simulink model "Demo_veDYNA_cs"  (Simulink 7.6)
settings: Solver=ode1  StartTime=0  StopTime=15  FixedStep=1/500  RelTol=1e-3
PreLoadFcn:
  | PreScanveDYNAPreLoadFcn(bdroot);
  | check_NUTS_defined;
  | 
  | assignin('base',['model_closed_' bdroot],false);
PostLoadFcn:
  | PreScanveDYNAPostLoadFcn(bdroot);
  | 
InitFcn:
  | vdy_SetExternalInputSource('ManLongCtrl',1,'Brake','other');
  | vdy_SetExternalInputSource('ManLongCtrl',1,'EngineTorque','other');
  | vdy_SetExternalInputSource('ManLatCtrl',1,'Steering','other');
  | 
  | PreScanveDYNAInitFcn(bdroot);
  | PreScanExperimentInitFcn(bdroot)
StopFcn:
  | PreScanExperimentStopFcn(bdroot)
undefined symbols (not defined in the file): at_period, CPT, vm_at_pulsewidth, vm_driver_dflt_gain, x_ini_VRML, y_ini_VRML, z_ini_VRML
libraries: dyna_cpt_lib x93, simulink x16, simulink_extras x14, PreScanSimulinkLibrary x6, anilib x3, dyna_lib x3, dyna_manctrl_lib x2, dyna_road_lib x2, PreScanUsefulBlocks x1, dyna_io_lib x1, dyna_demo_lib x1, dyna_usr_maneuver_states_lib x1
(part 7 of 8)

== system Demo_veDYNA_cs/Vedyna_Vehicle/CPT_MDL/MDL_PAR/Driver/System Instance 1/front_stiff [N/rad] ==
  Table : Lookup  InputValues=CPT.MDL_PAR.Driver{1}.front_stiff.Table.x  Table=CPT.MDL_PAR.Driver{1}.front_stiff.Table.v  SaturateOnIntegerOverflow=on
  Terminator : Terminator
  Terminator1 : Terminator
  Value : Constant  Value=CPT.MDL_PAR.Driver{1}.front_stiff.Value.v
  tag scope: Driver_1_front_stiff_TBL=global, Driver_1_front_stiff_VAL=global
  wires:
  [vdy_Simctrl_tsim] -> Table/1
  Value/1 -> [Driver_1_front_stiff_VAL]
  [Driver_1_front_stiff_VAL] -> Terminator/1
  [Driver_1_front_stiff_TBL] -> Terminator1/1
  Table/1 -> [Driver_1_front_stiff_TBL]

== system Demo_veDYNA_cs/Vedyna_Vehicle/CPT_MDL/MDL_PAR/Driver/System Instance 1/front_stiff_sw [-] ==
  Table : Lookup  InputValues=CPT.MDL_PAR.Driver{1}.front_stiff_sw.Table.x  Table=CPT.MDL_PAR.Driver{1}.front_stiff_sw.Table.v  SaturateOnIntegerOverflow=on
  Terminator : Terminator
  Terminator1 : Terminator
  Value : Constant  Value=CPT.MDL_PAR.Driver{1}.front_stiff_sw.Value.v
  tag scope: Driver_1_front_stiff_sw_TBL=global, Driver_1_front_stiff_sw_VAL=global
  wires:
  [vdy_Simctrl_tsim] -> Table/1
  Value/1 -> [Driver_1_front_stiff_sw_VAL]
  [Driver_1_front_stiff_sw_VAL] -> Terminator/1
  [Driver_1_front_stiff_sw_TBL] -> Terminator1/1
  Table/1 -> [Driver_1_front_stiff_sw_TBL]

== system Demo_veDYNA_cs/Vedyna_Vehicle/CPT_MDL/MDL_PAR/Driver/System Instance 1/gain_lat [-] ==
  Table : Lookup  InputValues=CPT.MDL_PAR.Driver{1}.gain_lat.Table.x  Table=CPT.MDL_PAR.Driver{1}.gain_lat.Table.v  SaturateOnIntegerOverflow=on
  Terminator : Terminator
  Terminator1 : Terminator
  Value : Constant  Value=CPT.MDL_PAR.Driver{1}.gain_lat.Value.v
  tag scope: Driver_1_gain_lat_TBL=global, Driver_1_gain_lat_VAL=global
  wires:
  [vdy_Simctrl_tsim] -> Table/1
  Value/1 -> [Driver_1_gain_lat_VAL]
  [Driver_1_gain_lat_VAL] -> Terminator/1
  [Driver_1_gain_lat_TBL] -> Terminator1/1
  Table/1 -> [Driver_1_gain_lat_TBL]

== system Demo_veDYNA_cs/Vedyna_Vehicle/CPT_MDL/MDL_PAR/Driver/System Instance 1/gain_long [-] ==
  Table : Lookup  InputValues=CPT.MDL_PAR.Driver{1}.gain_long.Table.x  Table=CPT.MDL_PAR.Driver{1}.gain_long.Table.v  SaturateOnIntegerOverflow=on
  Terminator : Terminator
  Terminator1 : Terminator
  Value : Constant  Value=CPT.MDL_PAR.Driver{1}.gain_long.Value.v
  tag scope: Driver_1_gain_long_TBL=global, Driver_1_gain_long_VAL=global
  wires:
  [vdy_Simctrl_tsim] -> Table/1
  Value/1 -> [Driver_1_gain_long_VAL]
  [Driver_1_gain_long_VAL] -> Terminator/1
  [Driver_1_gain_long_TBL] -> Terminator1/1
  Table/1 -> [Driver_1_gain_long_TBL]

== system Demo_veDYNA_cs/Vedyna_Vehicle/CPT_MDL/MDL_PAR/Driver/System Instance 1/lat_for_r_scale [-] ==
  Table : Lookup  InputValues=CPT.MDL_PAR.Driver{1}.lat_for_r_scale.Table.x  Table=CPT.MDL_PAR.Driver{1}.lat_for_r_scale.Table.v  SaturateOnIntegerOverflow=on
  Terminator : Terminator
  Terminator1 : Terminator
  Value : Constant  Value=CPT.MDL_PAR.Driver{1}.lat_for_r_scale.Value.v
  tag scope: Driver_1_lat_for_r_scale_TBL=global, Driver_1_lat_for_r_scale_VAL=global
  wires:
  [vdy_Simctrl_tsim] -> Table/1
  Value/1 -> [Driver_1_lat_for_r_scale_VAL]
  [Driver_1_lat_for_r_scale_VAL] -> Terminator/1
  [Driver_1_lat_for_r_scale_TBL] -> Terminator1/1
  Table/1 -> [Driver_1_lat_for_r_scale_TBL]

== system Demo_veDYNA_cs/Vedyna_Vehicle/CPT_MDL/MDL_PAR/Driver/System Instance 1/lat_for_r_smooth_t [s] ==
  Table : Lookup  InputValues=CPT.MDL_PAR.Driver{1}.lat_for_r_smooth_t.Table.x  Table=CPT.MDL_PAR.Driver{1}.lat_for_r_smooth_t.Table.v  SaturateOnIntegerOverflow=on
  Terminator : Terminator
  Terminator1 : Terminator
  Value : Constant  Value=CPT.MDL_PAR.Driver{1}.lat_for_r_smooth_t.Value.v
  tag scope: Driver_1_lat_for_r_smooth_t_TBL=global, Driver_1_lat_for_r_smooth_t_VAL=global
  wires:
  [vdy_Simctrl_tsim] -> Table/1
  Value/1 -> [Driver_1_lat_for_r_smooth_t_VAL]
  [Driver_1_lat_for_r_smooth_t_VAL] -> Terminator/1
  [Driver_1_lat_for_r_smooth_t_TBL] -> Terminator1/1
  Table/1 -> [Driver_1_lat_for_r_smooth_t_TBL]

== system Demo_veDYNA_cs/Vedyna_Vehicle/CPT_MDL/MDL_PAR/Driver/System Instance 1/lat_for_r_sw [-] ==
  Table : Lookup  InputValues=CPT.MDL_PAR.Driver{1}.lat_for_r_sw.Table.x  Table=CPT.MDL_PAR.Driver{1}.lat_for_r_sw.Table.v  SaturateOnIntegerOverflow=on
  Terminator : Terminator
  Terminator1 : Terminator
  Value : Constant  Value=CPT.MDL_PAR.Driver{1}.lat_for_r_sw.Value.v
  tag scope: Driver_1_lat_for_r_sw_TBL=global, Driver_1_lat_for_r_sw_VAL=global
  wires:
  [vdy_Simctrl_tsim] -> Table/1
  Value/1 -> [Driver_1_lat_for_r_sw_VAL]
  [Driver_1_lat_for_r_sw_VAL] -> Terminator/1
  [Driver_1_lat_for_r_sw_TBL] -> Terminator1/1
  Table/1 -> [Driver_1_lat_for_r_sw_TBL]

== system Demo_veDYNA_cs/Vedyna_Vehicle/CPT_MDL/MDL_PAR/Driver/System Instance 1/path_v_scale [-] ==
  Table : Lookup  InputValues=CPT.MDL_PAR.Driver{1}.path_v_scale.Table.x  Table=CPT.MDL_PAR.Driver{1}.path_v_scale.Table.v  SaturateOnIntegerOverflow=on
  Terminator : Terminator
  Terminator1 : Terminator
  Value : Constant  Value=CPT.MDL_PAR.Driver{1}.path_v_scale.Value.v
  tag scope: Driver_1_path_v_scale_TBL=global, Driver_1_path_v_scale_VAL=global
  wires:
  [vdy_Simctrl_tsim] -> Table/1
  Value/1 -> [Driver_1_path_v_scale_VAL]
  [Driver_1_path_v_scale_VAL] -> Terminator/1
  [Driver_1_path_v_scale_TBL] -> Terminator1/1
  Table/1 -> [Driver_1_path_v_scale_TBL]

== system Demo_veDYNA_cs/Vedyna_Vehicle/CPT_MDL/MDL_PAR/Driver/System Instance 1/path_x_offset [m] ==
  Table : Lookup  InputValues=CPT.MDL_PAR.Driver{1}.path_x_offset.Table.x  Table=CPT.MDL_PAR.Driver{1}.path_x_offset.Table.v  SaturateOnIntegerOverflow=on
  Terminator : Terminator
  Terminator1 : Terminator
  Value : Constant  Value=CPT.MDL_PAR.Driver{1}.path_x_offset.Value.v
  tag scope: Driver_1_path_x_offset_TBL=global, Driver_1_path_x_offset_VAL=global
  wires:
  [vdy_Simctrl_tsim] -> Table/1
  Value/1 -> [Driver_1_path_x_offset_VAL]
  [Driver_1_path_x_offset_VAL] -> Terminator/1
  [Driver_1_path_x_offset_TBL] -> Terminator1/1
  Table/1 -> [Driver_1_path_x_offset_TBL]

== system Demo_veDYNA_cs/Vedyna_Vehicle/CPT_MDL/MDL_PAR/Driver/System Instance 1/psi_path [rad] ==
  Table : Lookup  InputValues=CPT.MDL_PAR.Driver{1}.psi_path.Table.x  Table=CPT.MDL_PAR.Driver{1}.psi_path.Table.v  SaturateOnIntegerOverflow=on
  Terminator : Terminator
  Terminator1 : Terminator
  Value : Constant  Value=CPT.MDL_PAR.Driver{1}.psi_path.Value.v
  tag scope: Driver_1_psi_path_TBL=global, Driver_1_psi_path_VAL=global
  wires:
  [vdy_Driver_s] -> Table/1
  Value/1 -> [Driver_1_psi_path_VAL]
  [Driver_1_psi_path_VAL] -> Terminator/1
  [Driver_1_psi_path_TBL] -> Terminator1/1
  Table/1 -> [Driver_1_psi_path_TBL]

== system Demo_veDYNA_cs/Vedyna_Vehicle/CPT_MDL/MDL_PAR/Driver/System Instance 1/q_path [m] ==
  Table : Lookup  InputValues=CPT.MDL_PAR.Driver{1}.q_path.Table.x  Table=CPT.MDL_PAR.Driver{1}.q_path.Table.v  SaturateOnIntegerOverflow=on
  Terminator : Terminator
  Terminator1 : Terminator
  Value : Constant  Value=CPT.MDL_PAR.Driver{1}.q_path.Value.v
  tag scope: Driver_1_q_path_TBL=global, Driver_1_q_path_VAL=global
  wires:
  [vdy_Driver_s] -> Table/1
  Value/1 -> [Driver_1_q_path_VAL]
  [Driver_1_q_path_VAL] -> Terminator/1
  [Driver_1_q_path_TBL] -> Terminator1/1
  Table/1 -> [Driver_1_q_path_TBL]

== system Demo_veDYNA_cs/Vedyna_Vehicle/CPT_MDL/MDL_PAR/Driver/System Instance 1/rear_stiff [N/rad] ==
  Table : Lookup  InputValues=CPT.MDL_PAR.Driver{1}.rear_stiff.Table.x  Table=CPT.MDL_PAR.Driver{1}.rear_stiff.Table.v  SaturateOnIntegerOverflow=on
  Terminator : Terminator
  Terminator1 : Terminator
  Value : Constant  Value=CPT.MDL_PAR.Driver{1}.rear_stiff.Value.v
  tag scope: Driver_1_rear_stiff_TBL=global, Driver_1_rear_stiff_VAL=global
  wires:
  [vdy_Simctrl_tsim] -> Table/1
  Value/1 -> [Driver_1_rear_stiff_VAL]
  [Driver_1_rear_stiff_VAL] -> Terminator/1
  [Driver_1_rear_stiff_TBL] -> Terminator1/1
  Table/1 -> [Driver_1_rear_stiff_TBL]

== system Demo_veDYNA_cs/Vedyna_Vehicle/CPT_MDL/MDL_PAR/Driver/System Instance 1/rear_stiff_sw [-] ==
  Table : Lookup  InputValues=CPT.MDL_PAR.Driver{1}.rear_stiff_sw.Table.x  Table=CPT.MDL_PAR.Driver{1}.rear_stiff_sw.Table.v  SaturateOnIntegerOverflow=on
  Terminator : Terminator
  Terminator1 : Terminator
  Value : Constant  Value=CPT.MDL_PAR.Driver{1}.rear_stiff_sw.Value.v
  tag scope: Driver_1_rear_stiff_sw_TBL=global, Driver_1_rear_stiff_sw_VAL=global
  wires:
  [vdy_Simctrl_tsim] -> Table/1
  Value/1 -> [Driver_1_rear_stiff_sw_VAL]
  [Driver_1_rear_stiff_sw_VAL] -> Terminator/1
  [Driver_1_rear_stiff_sw_TBL] -> Terminator1/1
  Table/1 -> [Driver_1_rear_stiff_sw_TBL]

== system Demo_veDYNA_cs/Vedyna_Vehicle/CPT_MDL/MDL_PAR/Driver/System Instance 1/steer_max [deg] ==
  Table : Lookup  InputValues=CPT.MDL_PAR.Driver{1}.steer_max.Table.x  Table=CPT.MDL_PAR.Driver{1}.steer_max.Table.v  SaturateOnIntegerOverflow=on
  Terminator : Terminator
  Terminator1 : Terminator
  Value : Constant  Value=CPT.MDL_PAR.Driver{1}.steer_max.Value.v
  tag scope: Driver_1_steer_max_TBL=global, Driver_1_steer_max_VAL=global
  wires:
  [vdy_Simctrl_tsim] -> Table/1
  Value/1 -> [Driver_1_steer_max_VAL]
  [Driver_1_steer_max_VAL] -> Terminator/1
  [Driver_1_steer_max_TBL] -> Terminator1/1
  Table/1 -> [Driver_1_steer_max_TBL]

== system Demo_veDYNA_cs/Vedyna_Vehicle/CPT_MDL/MDL_PAR/Driver/System Instance 1/steer_min [deg] ==
  Table : Lookup  InputValues=CPT.MDL_PAR.Driver{1}.steer_min.Table.x  Table=CPT.MDL_PAR.Driver{1}.steer_min.Table.v  SaturateOnIntegerOverflow=on
  Terminator : Terminator
  Terminator1 : Terminator
  Value : Constant  Value=CPT.MDL_PAR.Driver{1}.steer_min.Value.v
  tag scope: Driver_1_steer_min_TBL=global, Driver_1_steer_min_VAL=global
  wires:
  [vdy_Simctrl_tsim] -> Table/1
  Value/1 -> [Driver_1_steer_min_VAL]
  [Driver_1_steer_min_VAL] -> Terminator/1
  [Driver_1_steer_min_TBL] -> Terminator1/1
  Table/1 -> [Driver_1_steer_min_TBL]

== system Demo_veDYNA_cs/Vedyna_Vehicle/CPT_MDL/MDL_PAR/Driver/System Instance 1/steer_rate_max [deg/s] ==
  Table : Lookup  InputValues=CPT.MDL_PAR.Driver{1}.steer_rate_max.Table.x  Table=CPT.MDL_PAR.Driver{1}.steer_rate_max.Table.v  SaturateOnIntegerOverflow=on
  Terminator : Terminator
  Terminator1 : Terminator
  Value : Constant  Value=CPT.MDL_PAR.Driver{1}.steer_rate_max.Value.v
  tag scope: Driver_1_steer_rate_max_TBL=global, Driver_1_steer_rate_max_VAL=global
  wires:
  [vdy_Simctrl_tsim] -> Table/1
  Value/1 -> [Driver_1_steer_rate_max_VAL]
  [Driver_1_steer_rate_max_VAL] -> Terminator/1
  [Driver_1_steer_rate_max_TBL] -> Terminator1/1
  Table/1 -> [Driver_1_steer_rate_max_TBL]

== system Demo_veDYNA_cs/Vedyna_Vehicle/CPT_MDL/MDL_PAR/Driver/System Instance 1/steer_rate_min [deg/s] ==
  Table : Lookup  InputValues=CPT.MDL_PAR.Driver{1}.steer_rate_min.Table.x  Table=CPT.MDL_PAR.Driver{1}.steer_rate_min.Table.v  SaturateOnIntegerOverflow=on
  Terminator : Terminator
  Terminator1 : Terminator
  Value : Constant  Value=CPT.MDL_PAR.Driver{1}.steer_rate_min.Value.v
  tag scope: Driver_1_steer_rate_min_TBL=global, Driver_1_steer_rate_min_VAL=global
  wires:
  [vdy_Simctrl_tsim] -> Table/1
  Value/1 -> [Driver_1_steer_rate_min_VAL]
  [Driver_1_steer_rate_min_VAL] -> Terminator/1
  [Driver_1_steer_rate_min_TBL] -> Terminator1/1
  Table/1 -> [Driver_1_steer_rate_min_TBL]

== system Demo_veDYNA_cs/Vedyna_Vehicle/CPT_MDL/MDL_PAR/Driver/System Instance 1/steer_smooth_t [s] ==
  Table : Lookup  InputValues=CPT.MDL_PAR.Driver{1}.steer_smooth_t.Table.x  Table=CPT.MDL_PAR.Driver{1}.steer_smooth_t.Table.v  SaturateOnIntegerOverflow=on
  Terminator : Terminator
  Terminator1 : Terminator
  Value : Constant  Value=CPT.MDL_PAR.Driver{1}.steer_smooth_t.Value.v
  tag scope: Driver_1_steer_smooth_t_TBL=global, Driver_1_steer_smooth_t_VAL=global
  wires:
  [vdy_Simctrl_tsim] -> Table/1
  Value/1 -> [Driver_1_steer_smooth_t_VAL]
  [Driver_1_steer_smooth_t_VAL] -> Terminator/1
  [Driver_1_steer_smooth_t_TBL] -> Terminator1/1
  Table/1 -> [Driver_1_steer_smooth_t_TBL]

== system Demo_veDYNA_cs/Vedyna_Vehicle/CPT_MDL/MDL_PAR/Driver/System Instance 1/target_aim_x [m] ==
  Table : Lookup  InputValues=CPT.MDL_PAR.Driver{1}.target_aim_x.Table.x  Table=CPT.MDL_PAR.Driver{1}.target_aim_x.Table.v  SaturateOnIntegerOverflow=on
  Terminator : Terminator
  Terminator1 : Terminator
  Value : Constant  Value=CPT.MDL_PAR.Driver{1}.target_aim_x.Value.v
  tag scope: Driver_1_target_aim_x_TBL=global, Driver_1_target_aim_x_VAL=global
  wires:
  [vdy_Simctrl_tsim] -> Table/1
  Value/1 -> [Driver_1_target_aim_x_VAL]
  [Driver_1_target_aim_x_VAL] -> Terminator/1
  [Driver_1_target_aim_x_TBL] -> Terminator1/1
  Table/1 -> [Driver_1_target_aim_x_TBL]

== system Demo_veDYNA_cs/Vedyna_Vehicle/CPT_MDL/MDL_PAR/Driver/System Instance 1/tgt_a_max [m/s^2] ==
  Table : Lookup  InputValues=CPT.MDL_PAR.Driver{1}.tgt_a_max.Table.x  Table=CPT.MDL_PAR.Driver{1}.tgt_a_max.Table.v  SaturateOnIntegerOverflow=on
  Terminator : Terminator
  Terminator1 : Terminator
  Value : Constant  Value=CPT.MDL_PAR.Driver{1}.tgt_a_max.Value.v
  tag scope: Driver_1_tgt_a_max_TBL=global, Driver_1_tgt_a_max_VAL=global
  wires:
  [vdy_Simctrl_tsim] -> Table/1
  Value/1 -> [Driver_1_tgt_a_max_VAL]
  [Driver_1_tgt_a_max_VAL] -> Terminator/1
  [Driver_1_tgt_a_max_TBL] -> Terminator1/1
  Table/1 -> [Driver_1_tgt_a_max_TBL]

== system Demo_veDYNA_cs/Vedyna_Vehicle/CPT_MDL/MDL_PAR/Driver/System Instance 1/tgt_acc_smooth_t [s] ==
  Table : Lookup  InputValues=CPT.MDL_PAR.Driver{1}.tgt_acc_smooth_t.Table.x  Table=CPT.MDL_PAR.Driver{1}.tgt_acc_smooth_t.Table.v  SaturateOnIntegerOverflow=on
  Terminator : Terminator
  Terminator1 : Terminator
  Value : Constant  Value=CPT.MDL_PAR.Driver{1}.tgt_acc_smooth_t.Value.v
  tag scope: Driver_1_tgt_acc_smooth_t_TBL=global, Driver_1_tgt_acc_smooth_t_VAL=global
  wires:
  [vdy_Simctrl_tsim] -> Table/1
  Value/1 -> [Driver_1_tgt_acc_smooth_t_VAL]
  [Driver_1_tgt_acc_smooth_t_VAL] -> Terminator/1
  [Driver_1_tgt_acc_smooth_t_TBL] -> Terminator1/1
  Table/1 -> [Driver_1_tgt_acc_smooth_t_TBL]

== system Demo_veDYNA_cs/Vedyna_Vehicle/CPT_MDL/MDL_PAR/Driver/System Instance 1/tgt_ax_max [m/s^2] ==
  Table : Lookup  InputValues=CPT.MDL_PAR.Driver{1}.tgt_ax_max.Table.x  Table=CPT.MDL_PAR.Driver{1}.tgt_ax_max.Table.v  SaturateOnIntegerOverflow=on
  Terminator : Terminator
  Terminator1 : Terminator
  Value : Constant  Value=CPT.MDL_PAR.Driver{1}.tgt_ax_max.Value.v
  tag scope: Driver_1_tgt_ax_max_TBL=global, Driver_1_tgt_ax_max_VAL=global
  wires:
  [vdy_Simctrl_tsim] -> Table/1
  Value/1 -> [Driver_1_tgt_ax_max_VAL]
  [Driver_1_tgt_ax_max_VAL] -> Terminator/1
  [Driver_1_tgt_ax_max_TBL] -> Terminator1/1
  Table/1 -> [Driver_1_tgt_ax_max_TBL]

== system Demo_veDYNA_cs/Vedyna_Vehicle/CPT_MDL/MDL_PAR/Driver/System Instance 1/tgt_ax_min [m/s^2] ==
  Table : Lookup  InputValues=CPT.MDL_PAR.Driver{1}.tgt_ax_min.Table.x  Table=CPT.MDL_PAR.Driver{1}.tgt_ax_min.Table.v  SaturateOnIntegerOverflow=on
  Terminator : Terminator
  Terminator1 : Terminator
  Value : Constant  Value=CPT.MDL_PAR.Driver{1}.tgt_ax_min.Value.v
  tag scope: Driver_1_tgt_ax_min_TBL=global, Driver_1_tgt_ax_min_VAL=global
  wires:
  [vdy_Simctrl_tsim] -> Table/1
  Value/1 -> [Driver_1_tgt_ax_min_VAL]
  [Driver_1_tgt_ax_min_VAL] -> Terminator/1
  [Driver_1_tgt_ax_min_TBL] -> Terminator1/1
  Table/1 -> [Driver_1_tgt_ax_min_TBL]

== system Demo_veDYNA_cs/Vedyna_Vehicle/CPT_MDL/MDL_PAR/Driver/System Instance 1/tgt_ay_max [m/s^2] ==
  Table : Lookup  InputValues=CPT.MDL_PAR.Driver{1}.tgt_ay_max.Table.x  Table=CPT.MDL_PAR.Driver{1}.tgt_ay_max.Table.v  SaturateOnIntegerOverflow=on
  Terminator : Terminator
  Terminator1 : Terminator
  Value : Constant  Value=CPT.MDL_PAR.Driver{1}.tgt_ay_max.Value.v
  tag scope: Driver_1_tgt_ay_max_TBL=global, Driver_1_tgt_ay_max_VAL=global
  wires:
  [vdy_Simctrl_tsim] -> Table/1
  Value/1 -> [Driver_1_tgt_ay_max_VAL]
  [Driver_1_tgt_ay_max_VAL] -> Terminator/1
  [Driver_1_tgt_ay_max_TBL] -> Terminator1/1
  Table/1 -> [Driver_1_tgt_ay_max_TBL]

== system Demo_veDYNA_cs/Vedyna_Vehicle/CPT_MDL/MDL_PAR/Driver/System Instance 1/tgt_v_max [m/s] ==
  Table : Lookup  InputValues=CPT.MDL_PAR.Driver{1}.tgt_v_max.Table.x  Table=CPT.MDL_PAR.Driver{1}.tgt_v_max.Table.v  SaturateOnIntegerOverflow=on
  Terminator : Terminator
  Terminator1 : Terminator
  Value : Constant  Value=CPT.MDL_PAR.Driver{1}.tgt_v_max.Value.v
  tag scope: Driver_1_tgt_v_max_TBL=global, Driver_1_tgt_v_max_VAL=global
  wires:
  [vdy_Simctrl_tsim] -> Table/1
  Value/1 -> [Driver_1_tgt_v_max_VAL]
  [Driver_1_tgt_v_max_VAL] -> Terminator/1
  [Driver_1_tgt_v_max_TBL] -> Terminator1/1
  Table/1 -> [Driver_1_tgt_v_max_TBL]

== system Demo_veDYNA_cs/Vedyna_Vehicle/CPT_MDL/MDL_PAR/Driver/System Instance 1/tgt_v_min [m/s] ==
  Table : Lookup  InputValues=CPT.MDL_PAR.Driver{1}.tgt_v_min.Table.x  Table=CPT.MDL_PAR.Driver{1}.tgt_v_min.Table.v  SaturateOnIntegerOverflow=on
  Terminator : Terminator
  Terminator1 : Terminator
  Value : Constant  Value=CPT.MDL_PAR.Driver{1}.tgt_v_min.Value.v
  tag scope: Driver_1_tgt_v_min_TBL=global, Driver_1_tgt_v_min_VAL=global
  wires:
  [vdy_Simctrl_tsim] -> Table/1
  Value/1 -> [Driver_1_tgt_v_min_VAL]
  [Driver_1_tgt_v_min_VAL] -> Terminator/1
  [Driver_1_tgt_v_min_TBL] -> Terminator1/1
  Table/1 -> [Driver_1_tgt_v_min_TBL]

== system Demo_veDYNA_cs/Vedyna_Vehicle/CPT_MDL/MDL_PAR/Driver/System Instance 1/use_simulink_sw [-] ==
  Table : Lookup  InputValues=CPT.MDL_PAR.Driver{1}.use_simulink_sw.Table.x  Table=CPT.MDL_PAR.Driver{1}.use_simulink_sw.Table.v  SaturateOnIntegerOverflow=on
  Terminator : Terminator
  Terminator1 : Terminator
  Value : Constant  Value=CPT.MDL_PAR.Driver{1}.use_simulink_sw.Value.v
  tag scope: Driver_1_use_simulink_sw_TBL=global, Driver_1_use_simulink_sw_VAL=global
  wires:
  [vdy_Simctrl_tsim] -> Table/1
  Value/1 -> [Driver_1_use_simulink_sw_VAL]
  [Driver_1_use_simulink_sw_VAL] -> Terminator/1
  [Driver_1_use_simulink_sw_TBL] -> Terminator1/1
  Table/1 -> [Driver_1_use_simulink_sw_TBL]

== system Demo_veDYNA_cs/Vedyna_Vehicle/CPT_MDL/MDL_PAR/Driver/System Instance 1/v_comp_scale [-] ==
  Table : Lookup  InputValues=CPT.MDL_PAR.Driver{1}.v_comp_scale.Table.x  Table=CPT.MDL_PAR.Driver{1}.v_comp_scale.Table.v  SaturateOnIntegerOverflow=on
  Terminator : Terminator
  Terminator1 : Terminator
  Value : Constant  Value=CPT.MDL_PAR.Driver{1}.v_comp_scale.Value.v
  tag scope: Driver_1_v_comp_scale_TBL=global, Driver_1_v_comp_scale_VAL=global
  wires:
  [vdy_Simctrl_tsim] -> Table/1
  Value/1 -> [Driver_1_v_comp_scale_VAL]
  [Driver_1_v_comp_scale_VAL] -> Terminator/1
  [Driver_1_v_comp_scale_TBL] -> Terminator1/1
  Table/1 -> [Driver_1_v_comp_scale_TBL]

== system Demo_veDYNA_cs/Vedyna_Vehicle/CPT_MDL/MDL_PAR/Driver/System Instance 1/v_path [m/s] ==
  Table : Lookup  InputValues=CPT.MDL_PAR.Driver{1}.v_path.Table.x  Table=CPT.MDL_PAR.Driver{1}.v_path.Table.v  SaturateOnIntegerOverflow=on
  Terminator : Terminator
  Terminator1 : Terminator
  Value : Constant  Value=CPT.MDL_PAR.Driver{1}.v_path.Value.v
  tag scope: Driver_1_v_path_TBL=global, Driver_1_v_path_VAL=global
  wires:
  [vdy_Simctrl_tsim] -> Table/1
  Value/1 -> [Driver_1_v_path_VAL]
  [Driver_1_v_path_VAL] -> Terminator/1
  [Driver_1_v_path_TBL] -> Terminator1/1
  Table/1 -> [Driver_1_v_path_TBL]

== system Demo_veDYNA_cs/Vedyna_Vehicle/CPT_MDL/MDL_PAR/Engine/System Instance 1/ASR_Flag [-] ==
  Table : Lookup  InputValues=CPT.MDL_PAR.Engine{1}.ASR_Flag.Table.x  Table=CPT.MDL_PAR.Engine{1}.ASR_Flag.Table.v  SaturateOnIntegerOverflow=on
  Terminator : Terminator
  Terminator1 : Terminator
  Value : Constant  Value=CPT.MDL_PAR.Engine{1}.ASR_Flag.Value.v
  tag scope: Engine_1_ASR_Flag_TBL=global, Engine_1_ASR_Flag_VAL=global
  wires:
  [vdy_Simctrl_tsim] -> Table/1
  Value/1 -> [Engine_1_ASR_Flag_VAL]
  [Engine_1_ASR_Flag_VAL] -> Terminator/1
  [Engine_1_ASR_Flag_TBL] -> Terminator1/1
  Table/1 -> [Engine_1_ASR_Flag_TBL]

== system Demo_veDYNA_cs/Vedyna_Vehicle/CPT_MDL/MDL_PAR/Engine/System Instance 1/ASR_Torque [Nm] ==
  Table : Lookup  InputValues=CPT.MDL_PAR.Engine{1}.ASR_Torque.Table.x  Table=CPT.MDL_PAR.Engine{1}.ASR_Torque.Table.v  SaturateOnIntegerOverflow=on
  Terminator : Terminator
  Terminator1 : Terminator
  Value : Constant  Value=CPT.MDL_PAR.Engine{1}.ASR_Torque.Value.v
  tag scope: Engine_1_ASR_Torque_TBL=global, Engine_1_ASR_Torque_VAL=global
  wires:
  [vdy_Simctrl_tsim] -> Table/1
  Value/1 -> [Engine_1_ASR_Torque_VAL]
  [Engine_1_ASR_Torque_VAL] -> Terminator/1
  [Engine_1_ASR_Torque_TBL] -> Terminator1/1
  Table/1 -> [Engine_1_ASR_Torque_TBL]

== system Demo_veDYNA_cs/Vedyna_Vehicle/CPT_MDL/MDL_PAR/Engine/System Instance 1/MSR_Flag [-] ==
  Table : Lookup  InputValues=CPT.MDL_PAR.Engine{1}.MSR_Flag.Table.x  Table=CPT.MDL_PAR.Engine{1}.MSR_Flag.Table.v  SaturateOnIntegerOverflow=on
  Terminator : Terminator
  Terminator1 : Terminator
  Value : Constant  Value=CPT.MDL_PAR.Engine{1}.MSR_Flag.Value.v
  tag scope: Engine_1_MSR_Flag_TBL=global, Engine_1_MSR_Flag_VAL=global
  wires:
  [vdy_Simctrl_tsim] -> Table/1
  Value/1 -> [Engine_1_MSR_Flag_VAL]
  [Engine_1_MSR_Flag_VAL] -> Terminator/1
  [Engine_1_MSR_Flag_TBL] -> Terminator1/1
  Table/1 -> [Engine_1_MSR_Flag_TBL]

== system Demo_veDYNA_cs/Vedyna_Vehicle/CPT_MDL/MDL_PAR/Engine/System Instance 1/MSR_Torque [Nm] ==
  Table : Lookup  InputValues=CPT.MDL_PAR.Engine{1}.MSR_Torque.Table.x  Table=CPT.MDL_PAR.Engine{1}.MSR_Torque.Table.v  SaturateOnIntegerOverflow=on
  Terminator : Terminator
  Terminator1 : Terminator
  Value : Constant  Value=CPT.MDL_PAR.Engine{1}.MSR_Torque.Value.v
  tag scope: Engine_1_MSR_Torque_TBL=global, Engine_1_MSR_Torque_VAL=global
  wires:
  [vdy_Simctrl_tsim] -> Table/1
  Value/1 -> [Engine_1_MSR_Torque_VAL]
  [Engine_1_MSR_Torque_VAL] -> Terminator/1
  [Engine_1_MSR_Torque_TBL] -> Terminator1/1
  Table/1 -> [Engine_1_MSR_Torque_TBL]

== system Demo_veDYNA_cs/Vedyna_Vehicle/CPT_MDL/MDL_PAR/GearCtrl/System Instance 1/Gear [-] ==
  Table : Lookup  InputValues=CPT.MDL_PAR.GearCtrl{1}.Gear.Table.x  Table=CPT.MDL_PAR.GearCtrl{1}.Gear.Table.v  SaturateOnIntegerOverflow=on
  Terminator : Terminator
  Terminator1 : Terminator
  Value : Constant  Value=CPT.MDL_PAR.GearCtrl{1}.Gear.Value.v
  tag scope: GearCtrl_1_Gear_TBL=global, GearCtrl_1_Gear_VAL=global
  wires:
  [vdy_Simctrl_tsim] -> Table/1
  Value/1 -> [GearCtrl_1_Gear_VAL]
  [GearCtrl_1_Gear_VAL] -> Terminator/1
  [GearCtrl_1_Gear_TBL] -> Terminator1/1
  Table/1 -> [GearCtrl_1_Gear_TBL]

== system Demo_veDYNA_cs/Vedyna_Vehicle/CPT_MDL/MDL_PAR/GearCtrl/System Instance 1/UpShiftRequest [-1,1] ==
  Table : Lookup  InputValues=CPT.MDL_PAR.GearCtrl{1}.UpShiftRequest.Table.x  Table=CPT.MDL_PAR.GearCtrl{1}.UpShiftRequest.Table.v  SaturateOnIntegerOverflow=on
  Terminator : Terminator
  Terminator1 : Terminator
  Value : Constant  Value=CPT.MDL_PAR.GearCtrl{1}.UpShiftRequest.Value.v
  tag scope: GearCtrl_1_UpShiftRequest_TBL=global, GearCtrl_1_UpShiftRequest_VAL=global
  wires:
  [vdy_Simctrl_tsim] -> Table/1
  Value/1 -> [GearCtrl_1_UpShiftRequest_VAL]
  [GearCtrl_1_UpShiftRequest_VAL] -> Terminator/1
  [GearCtrl_1_UpShiftRequest_TBL] -> Terminator1/1
  Table/1 -> [GearCtrl_1_UpShiftRequest_TBL]

== system Demo_veDYNA_cs/Vedyna_Vehicle/CPT_MDL/MDL_PAR/ManLatCtrl/System Instance 1/Curvature [1/m] ==
  Table : Lookup  InputValues=CPT.MDL_PAR.ManLatCtrl{1}.Curvature.Table.x  Table=CPT.MDL_PAR.ManLatCtrl{1}.Curvature.Table.v  SaturateOnIntegerOverflow=on
  Terminator : Terminator
  Terminator1 : Terminator
  Value : Constant  Value=CPT.MDL_PAR.ManLatCtrl{1}.Curvature.Value.v
  tag scope: ManLatCtrl_1_Curvature_TBL=global, ManLatCtrl_1_Curvature_VAL=global
  wires:
  [vdy_Simctrl_tsim] -> Table/1
  Value/1 -> [ManLatCtrl_1_Curvature_VAL]
  [ManLatCtrl_1_Curvature_VAL] -> Terminator/1
  [ManLatCtrl_1_Curvature_TBL] -> Terminator1/1
  Table/1 -> [ManLatCtrl_1_Curvature_TBL]

== system Demo_veDYNA_cs/Vedyna_Vehicle/CPT_MDL/MDL_PAR/ManLatCtrl/System Instance 1/Steering [deg] ==
  Table : Lookup  InputValues=CPT.MDL_PAR.ManLatCtrl{1}.Steering.Table.x  Table=CPT.MDL_PAR.ManLatCtrl{1}.Steering.Table.v  SaturateOnIntegerOverflow=on
  Terminator : Terminator
  Terminator1 : Terminator
  Value : Constant  Value=CPT.MDL_PAR.ManLatCtrl{1}.Steering.Value.v
  tag scope: ManLatCtrl_1_Steering_TBL=global, ManLatCtrl_1_Steering_VAL=global
  wires:
  [vdy_Simctrl_tsim] -> Table/1
  Value/1 -> [ManLatCtrl_1_Steering_VAL]
  [ManLatCtrl_1_Steering_VAL] -> Terminator/1
  [ManLatCtrl_1_Steering_TBL] -> Terminator1/1
  Table/1 -> [ManLatCtrl_1_Steering_TBL]

== system Demo_veDYNA_cs/Vedyna_Vehicle/CPT_MDL/MDL_PAR/ManLongCtrl/System Instance 1/AccelerationY [m/s**2] ==
  Table : Lookup  InputValues=CPT.MDL_PAR.ManLongCtrl{1}.AccelerationY.Table.x  Table=CPT.MDL_PAR.ManLongCtrl{1}.AccelerationY.Table.v  SaturateOnIntegerOverflow=on
  Terminator : Terminator
  Terminator1 : Terminator
  Value : Constant  Value=CPT.MDL_PAR.ManLongCtrl{1}.AccelerationY.Value.v
  tag scope: ManLongCtrl_1_AccelerationY_TBL=global, ManLongCtrl_1_AccelerationY_VAL=global
  wires:
  [vdy_Simctrl_tsim] -> Table/1
  Value/1 -> [ManLongCtrl_1_AccelerationY_VAL]
  [ManLongCtrl_1_AccelerationY_VAL] -> Terminator/1
  [ManLongCtrl_1_AccelerationY_TBL] -> Terminator1/1
  Table/1 -> [ManLongCtrl_1_AccelerationY_TBL]

== system Demo_veDYNA_cs/Vedyna_Vehicle/CPT_MDL/MDL_PAR/ManLongCtrl/System Instance 1/Brake [%] ==
  Table : Lookup  InputValues=CPT.MDL_PAR.ManLongCtrl{1}.Brake.Table.x  Table=CPT.MDL_PAR.ManLongCtrl{1}.Brake.Table.v  SaturateOnIntegerOverflow=on
  Terminator : Terminator
  Terminator1 : Terminator
  Value : Constant  Value=CPT.MDL_PAR.ManLongCtrl{1}.Brake.Value.v
  tag scope: ManLongCtrl_1_Brake_TBL=global, ManLongCtrl_1_Brake_VAL=global
  wires:
  [vdy_Simctrl_tsim] -> Table/1
  Value/1 -> [ManLongCtrl_1_Brake_VAL]
  [ManLongCtrl_1_Brake_VAL] -> Terminator/1
  [ManLongCtrl_1_Brake_TBL] -> Terminator1/1
  Table/1 -> [ManLongCtrl_1_Brake_TBL]

== system Demo_veDYNA_cs/Vedyna_Vehicle/CPT_MDL/MDL_PAR/ManLongCtrl/System Instance 1/EngineTorque [Nm] ==
  Table : Lookup  InputValues=CPT.MDL_PAR.ManLongCtrl{1}.EngineTorque.Table.x  Table=CPT.MDL_PAR.ManLongCtrl{1}.EngineTorque.Table.v  SaturateOnIntegerOverflow=on
  Terminator : Terminator
  Terminator1 : Terminator
  Value : Constant  Value=CPT.MDL_PAR.ManLongCtrl{1}.EngineTorque.Value.v
  tag scope: ManLongCtrl_1_EngineTorque_TBL=global, ManLongCtrl_1_EngineTorque_VAL=global
  wires:
  [vdy_Simctrl_tsim] -> Table/1
  Value/1 -> [ManLongCtrl_1_EngineTorque_VAL]
  [ManLongCtrl_1_EngineTorque_VAL] -> Terminator/1
  [ManLongCtrl_1_EngineTorque_TBL] -> Terminator1/1
  Table/1 -> [ManLongCtrl_1_EngineTorque_TBL]

== system Demo_veDYNA_cs/Vedyna_Vehicle/CPT_MDL/MDL_PAR/ManLongCtrl/System Instance 1/Speed [km/h] ==
  Table : Lookup  InputValues=CPT.MDL_PAR.ManLongCtrl{1}.Speed.Table.x  Table=CPT.MDL_PAR.ManLongCtrl{1}.Speed.Table.v  SaturateOnIntegerOverflow=on
  Terminator : Terminator
  Terminator1 : Terminator
  Value : Constant  Value=CPT.MDL_PAR.ManLongCtrl{1}.Speed.Value.v
  tag scope: ManLongCtrl_1_Speed_TBL=global, ManLongCtrl_1_Speed_VAL=global
  wires:
  [vdy_Simctrl_tsim] -> Table/1
  Value/1 -> [ManLongCtrl_1_Speed_VAL]
  [ManLongCtrl_1_Speed_VAL] -> Terminator/1
  [ManLongCtrl_1_Speed_TBL] -> Terminator1/1
  Table/1 -> [ManLongCtrl_1_Speed_TBL]

== system Demo_veDYNA_cs/Vedyna_Vehicle/CPT_MDL/MDL_PAR/ManLongCtrl/System Instance 1/Throttle [%] ==
  Table : Lookup  InputValues=CPT.MDL_PAR.ManLongCtrl{1}.Throttle.Table.x  Table=CPT.MDL_PAR.ManLongCtrl{1}.Throttle.Table.v  SaturateOnIntegerOverflow=on
  Terminator : Terminator
  Terminator1 : Terminator
  Value : Constant  Value=CPT.MDL_PAR.ManLongCtrl{1}.Throttle.Value.v
  tag scope: ManLongCtrl_1_Throttle_TBL=global, ManLongCtrl_1_Throttle_VAL=global
  wires:
  [vdy_Simctrl_tsim] -> Table/1
  Value/1 -> [ManLongCtrl_1_Throttle_VAL]
  [ManLongCtrl_1_Throttle_VAL] -> Terminator/1
  [ManLongCtrl_1_Throttle_TBL] -> Terminator1/1
  Table/1 -> [ManLongCtrl_1_Throttle_TBL]

== system Demo_veDYNA_cs/Vedyna_Vehicle/CPT_MDL/MDL_PAR/Tmeasy/System Instance 1/RoadMueScale [0..1] ==
  Table : Lookup  InputValues=CPT.MDL_PAR.Tmeasy{1}.RoadMueScale.Table.x  Table=CPT.MDL_PAR.Tmeasy{1}.RoadMueScale.Table.v  SaturateOnIntegerOverflow=on
  Terminator : Terminator
  Terminator1 : Terminator
  Value : Constant  Value=CPT.MDL_PAR.Tmeasy{1}.RoadMueScale.Value.v
  tag scope: Tmeasy_1_RoadMueScale_TBL=global, Tmeasy_1_RoadMueScale_VAL=global
  wires:
  [vdy_Simctrl_tsim] -> Table/1
  Value/1 -> [Tmeasy_1_RoadMueScale_VAL]
  [Tmeasy_1_RoadMueScale_VAL] -> Terminator/1
  [Tmeasy_1_RoadMueScale_TBL] -> Terminator1/1
  Table/1 -> [Tmeasy_1_RoadMueScale_TBL]

== system Demo_veDYNA_cs/Vedyna_Vehicle/CPT_MDL/MDL_PAR/Tmeasy/System Instance 2/RoadMueScale [0..1] ==
  Table : Lookup  InputValues=CPT.MDL_PAR.Tmeasy{2}.RoadMueScale.Table.x  Table=CPT.MDL_PAR.Tmeasy{2}.RoadMueScale.Table.v  SaturateOnIntegerOverflow=on
  Terminator : Terminator
  Terminator1 : Terminator
  Value : Constant  Value=CPT.MDL_PAR.Tmeasy{2}.RoadMueScale.Value.v
  tag scope: Tmeasy_2_RoadMueScale_TBL=global, Tmeasy_2_RoadMueScale_VAL=global
  wires:
  [vdy_Simctrl_tsim] -> Table/1
  Value/1 -> [Tmeasy_2_RoadMueScale_VAL]
  [Tmeasy_2_RoadMueScale_VAL] -> Terminator/1
  [Tmeasy_2_RoadMueScale_TBL] -> Terminator1/1
  Table/1 -> [Tmeasy_2_RoadMueScale_TBL]

== system Demo_veDYNA_cs/Vedyna_Vehicle/CPT_MDL/MDL_PAR/Tmeasy/System Instance 3/RoadMueScale [0..1] ==
  Table : Lookup  InputValues=CPT.MDL_PAR.Tmeasy{3}.RoadMueScale.Table.x  Table=CPT.MDL_PAR.Tmeasy{3}.RoadMueScale.Table.v  SaturateOnIntegerOverflow=on
  Terminator : Terminator
  Terminator1 : Terminator
  Value : Constant  Value=CPT.MDL_PAR.Tmeasy{3}.RoadMueScale.Value.v
  tag scope: Tmeasy_3_RoadMueScale_TBL=global, Tmeasy_3_RoadMueScale_VAL=global
  wires:
  [vdy_Simctrl_tsim] -> Table/1
  Value/1 -> [Tmeasy_3_RoadMueScale_VAL]
  [Tmeasy_3_RoadMueScale_VAL] -> Terminator/1
  [Tmeasy_3_RoadMueScale_TBL] -> Terminator1/1
  Table/1 -> [Tmeasy_3_RoadMueScale_TBL]

== system Demo_veDYNA_cs/Vedyna_Vehicle/CPT_MDL/MDL_PAR/Tmeasy/System Instance 4/RoadMueScale [0..1] ==
  Table : Lookup  InputValues=CPT.MDL_PAR.Tmeasy{4}.RoadMueScale.Table.x  Table=CPT.MDL_PAR.Tmeasy{4}.RoadMueScale.Table.v  SaturateOnIntegerOverflow=on
  Terminator : Terminator
  Terminator1 : Terminator
  Value : Constant  Value=CPT.MDL_PAR.Tmeasy{4}.RoadMueScale.Value.v
  tag scope: Tmeasy_4_RoadMueScale_TBL=global, Tmeasy_4_RoadMueScale_VAL=global
  wires:
  [vdy_Simctrl_tsim] -> Table/1
  Value/1 -> [Tmeasy_4_RoadMueScale_VAL]
  [Tmeasy_4_RoadMueScale_VAL] -> Terminator/1
  [Tmeasy_4_RoadMueScale_TBL] -> Terminator1/1
  Table/1 -> [Tmeasy_4_RoadMueScale_TBL]

== system Demo_veDYNA_cs/Vedyna_Vehicle/CPT_MDL/MDL_PAR/Tmeasy/System Instance 5/RoadMueScale [0..1] ==
  Table : Lookup  InputValues=CPT.MDL_PAR.Tmeasy{5}.RoadMueScale.Table.x  Table=CPT.MDL_PAR.Tmeasy{5}.RoadMueScale.Table.v  SaturateOnIntegerOverflow=on
  Terminator : Terminator
  Terminator1 : Terminator
  Value : Constant  Value=CPT.MDL_PAR.Tmeasy{5}.RoadMueScale.Value.v
  tag scope: Tmeasy_5_RoadMueScale_TBL=global, Tmeasy_5_RoadMueScale_VAL=global
  wires:
  [vdy_Simctrl_tsim] -> Table/1
  Value/1 -> [Tmeasy_5_RoadMueScale_VAL]
  [Tmeasy_5_RoadMueScale_VAL] -> Terminator/1
  [Tmeasy_5_RoadMueScale_TBL] -> Terminator1/1
  Table/1 -> [Tmeasy_5_RoadMueScale_TBL]

== system Demo_veDYNA_cs/Vedyna_Vehicle/CPT_MDL/MDL_PAR/Tmeasy/System Instance 6/RoadMueScale [0..1] ==
  Table : Lookup  InputValues=CPT.MDL_PAR.Tmeasy{6}.RoadMueScale.Table.x  Table=CPT.MDL_PAR.Tmeasy{6}.RoadMueScale.Table.v  SaturateOnIntegerOverflow=on
  Terminator : Terminator
  Terminator1 : Terminator
  Value : Constant  Value=CPT.MDL_PAR.Tmeasy{6}.RoadMueScale.Value.v
  tag scope: Tmeasy_6_RoadMueScale_TBL=global, Tmeasy_6_RoadMueScale_VAL=global
  wires:
  [vdy_Simctrl_tsim] -> Table/1
  Value/1 -> [Tmeasy_6_RoadMueScale_VAL]
  [Tmeasy_6_RoadMueScale_VAL] -> Terminator/1
  [Tmeasy_6_RoadMueScale_TBL] -> Terminator1/1
  Table/1 -> [Tmeasy_6_RoadMueScale_TBL]

== system Demo_veDYNA_cs/Vedyna_Vehicle/CPT_MDL/MDL_PAR/Tmeasy/System Instance 7/RoadMueScale [0..1] ==
  Table : Lookup  InputValues=CPT.MDL_PAR.Tmeasy{7}.RoadMueScale.Table.x  Table=CPT.MDL_PAR.Tmeasy{7}.RoadMueScale.Table.v  SaturateOnIntegerOverflow=on
  Terminator : Terminator
  Terminator1 : Terminator
  Value : Constant  Value=CPT.MDL_PAR.Tmeasy{7}.RoadMueScale.Value.v
  tag scope: Tmeasy_7_RoadMueScale_TBL=global, Tmeasy_7_RoadMueScale_VAL=global
  wires:
  Table/1 -> [Tmeasy_7_RoadMueScale_TBL]
  [Tmeasy_7_RoadMueScale_TBL] -> Terminator1/1
  [Tmeasy_7_RoadMueScale_VAL] -> Terminator/1
  Value/1 -> [Tmeasy_7_RoadMueScale_VAL]
  [vdy_Simctrl_tsim] -> Table/1

== system Demo_veDYNA_cs/Vedyna_Vehicle/CPT_MDL/MDL_PAR/Tmeasy/System Instance 8/RoadMueScale [0..1] ==
  Table : Lookup  InputValues=CPT.MDL_PAR.Tmeasy{8}.RoadMueScale.Table.x  Table=CPT.MDL_PAR.Tmeasy{8}.RoadMueScale.Table.v  SaturateOnIntegerOverflow=on
  Terminator : Terminator
  Terminator1 : Terminator
  Value : Constant  Value=CPT.MDL_PAR.Tmeasy{8}.RoadMueScale.Value.v
  tag scope: Tmeasy_8_RoadMueScale_TBL=global, Tmeasy_8_RoadMueScale_VAL=global
  wires:
  Table/1 -> [Tmeasy_8_RoadMueScale_TBL]
  [Tmeasy_8_RoadMueScale_TBL] -> Terminator1/1
  [Tmeasy_8_RoadMueScale_VAL] -> Terminator/1
  Value/1 -> [Tmeasy_8_RoadMueScale_VAL]
  [vdy_Simctrl_tsim] -> Table/1

== system Demo_veDYNA_cs/Vedyna_Vehicle/CPT_MDL/MDL_PAR/Wheel/System Instance 1/pbrm [N/m**2] ==
  Table : Lookup  InputValues=CPT.MDL_PAR.Wheel{1}.pbrm.Table.x  Table=CPT.MDL_PAR.Wheel{1}.pbrm.Table.v  SaturateOnIntegerOverflow=on
  Terminator : Terminator
  Terminator1 : Terminator
  Value : Constant  Value=CPT.MDL_PAR.Wheel{1}.pbrm.Value.v
  tag scope: Wheel_1_pbrm_TBL=global, Wheel_1_pbrm_VAL=global
  wires:
  [vdy_Simctrl_tsim] -> Table/1
  Value/1 -> [Wheel_1_pbrm_VAL]
  [Wheel_1_pbrm_VAL] -> Terminator/1
  [Wheel_1_pbrm_TBL] -> Terminator1/1
  Table/1 -> [Wheel_1_pbrm_TBL]

== system Demo_veDYNA_cs/Vedyna_Vehicle/CPT_MDL/MDL_PAR/Wheel/System Instance 2/pbrm [N/m**2] ==
  Table : Lookup  InputValues=CPT.MDL_PAR.Wheel{2}.pbrm.Table.x  Table=CPT.MDL_PAR.Wheel{2}.pbrm.Table.v  SaturateOnIntegerOverflow=on
  Terminator : Terminator
  Terminator1 : Terminator
  Value : Constant  Value=CPT.MDL_PAR.Wheel{2}.pbrm.Value.v
  tag scope: Wheel_2_pbrm_TBL=global, Wheel_2_pbrm_VAL=global
  wires:
  [vdy_Simctrl_tsim] -> Table/1
  Value/1 -> [Wheel_2_pbrm_VAL]
  [Wheel_2_pbrm_VAL] -> Terminator/1
  [Wheel_2_pbrm_TBL] -> Terminator1/1
  Table/1 -> [Wheel_2_pbrm_TBL]

== system Demo_veDYNA_cs/Vedyna_Vehicle/CPT_MDL/MDL_PAR/Wheel/System Instance 3/pbrm [N/m**2] ==
  Table : Lookup  InputValues=CPT.MDL_PAR.Wheel{3}.pbrm.Table.x  Table=CPT.MDL_PAR.Wheel{3}.pbrm.Table.v  SaturateOnIntegerOverflow=on
  Terminator : Terminator
  Terminator1 : Terminator
  Value : Constant  Value=CPT.MDL_PAR.Wheel{3}.pbrm.Value.v
  tag scope: Wheel_3_pbrm_TBL=global, Wheel_3_pbrm_VAL=global
  wires:
  [vdy_Simctrl_tsim] -> Table/1
  Value/1 -> [Wheel_3_pbrm_VAL]
  [Wheel_3_pbrm_VAL] -> Terminator/1
  [Wheel_3_pbrm_TBL] -> Terminator1/1
  Table/1 -> [Wheel_3_pbrm_TBL]

== system Demo_veDYNA_cs/Vedyna_Vehicle/CPT_MDL/MDL_PAR/Wheel/System Instance 4/pbrm [N/m**2] ==
  Table : Lookup  InputValues=CPT.MDL_PAR.Wheel{4}.pbrm.Table.x  Table=CPT.MDL_PAR.Wheel{4}.pbrm.Table.v  SaturateOnIntegerOverflow=on
  Terminator : Terminator
  Terminator1 : Terminator
  Value : Constant  Value=CPT.MDL_PAR.Wheel{4}.pbrm.Value.v
  tag scope: Wheel_4_pbrm_TBL=global, Wheel_4_pbrm_VAL=global
  wires:
  [vdy_Simctrl_tsim] -> Table/1
  Value/1 -> [Wheel_4_pbrm_VAL]
  [Wheel_4_pbrm_VAL] -> Terminator/1
  [Wheel_4_pbrm_TBL] -> Terminator1/1
  Table/1 -> [Wheel_4_pbrm_TBL]

== system Demo_veDYNA_cs/Vedyna_Vehicle/CPT_MDL/MDL_PAR/Wheel/System Instance 5/pbrm [N/m**2] ==
  Table : Lookup  InputValues=CPT.MDL_PAR.Wheel{5}.pbrm.Table.x  Table=CPT.MDL_PAR.Wheel{5}.pbrm.Table.v  SaturateOnIntegerOverflow=on
  Terminator : Terminator
  Terminator1 : Terminator
  Value : Constant  Value=CPT.MDL_PAR.Wheel{5}.pbrm.Value.v
  tag scope: Wheel_5_pbrm_TBL=global, Wheel_5_pbrm_VAL=global
  wires:
  [vdy_Simctrl_tsim] -> Table/1
  Value/1 -> [Wheel_5_pbrm_VAL]
  [Wheel_5_pbrm_VAL] -> Terminator/1
  [Wheel_5_pbrm_TBL] -> Terminator1/1
  Table/1 -> [Wheel_5_pbrm_TBL]

== system Demo_veDYNA_cs/Vedyna_Vehicle/CPT_MDL/MDL_PAR/Wheel/System Instance 6/pbrm [N/m**2] ==
  Table : Lookup  InputValues=CPT.MDL_PAR.Wheel{6}.pbrm.Table.x  Table=CPT.MDL_PAR.Wheel{6}.pbrm.Table.v  SaturateOnIntegerOverflow=on
  Terminator : Terminator
  Terminator1 : Terminator
  Value : Constant  Value=CPT.MDL_PAR.Wheel{6}.pbrm.Value.v
  tag scope: Wheel_6_pbrm_TBL=global, Wheel_6_pbrm_VAL=global
  wires:
  [vdy_Simctrl_tsim] -> Table/1
  Value/1 -> [Wheel_6_pbrm_VAL]
  [Wheel_6_pbrm_VAL] -> Terminator/1
  [Wheel_6_pbrm_TBL] -> Terminator1/1
  Table/1 -> [Wheel_6_pbrm_TBL]

== system Demo_veDYNA_cs/Vedyna_Vehicle/CPT_MDL/MDL_PAR/Wheel/System Instance 7/pbrm [N/m**2] ==
  Table : Lookup  InputValues=CPT.MDL_PAR.Wheel{7}.pbrm.Table.x  Table=CPT.MDL_PAR.Wheel{7}.pbrm.Table.v  SaturateOnIntegerOverflow=on
  Terminator : Terminator
  Terminator1 : Terminator
  Value : Constant  Value=CPT.MDL_PAR.Wheel{7}.pbrm.Value.v
  tag scope: Wheel_7_pbrm_TBL=global, Wheel_7_pbrm_VAL=global
  wires:
  Table/1 -> [Wheel_7_pbrm_TBL]
  [Wheel_7_pbrm_TBL] -> Terminator1/1
  [Wheel_7_pbrm_VAL] -> Terminator/1
  Value/1 -> [Wheel_7_pbrm_VAL]
  [vdy_Simctrl_tsim] -> Table/1

== system Demo_veDYNA_cs/Vedyna_Vehicle/CPT_MDL/MDL_PAR/Wheel/System Instance 8/pbrm [N/m**2] ==
  Table : Lookup  InputValues=CPT.MDL_PAR.Wheel{8}.pbrm.Table.x  Table=CPT.MDL_PAR.Wheel{8}.pbrm.Table.v  SaturateOnIntegerOverflow=on
  Terminator : Terminator
  Terminator1 : Terminator
  Value : Constant  Value=CPT.MDL_PAR.Wheel{8}.pbrm.Value.v
  tag scope: Wheel_8_pbrm_TBL=global, Wheel_8_pbrm_VAL=global
  wires:
  Table/1 -> [Wheel_8_pbrm_TBL]
  [Wheel_8_pbrm_TBL] -> Terminator1/1
  [Wheel_8_pbrm_VAL] -> Terminator/1
  Value/1 -> [Wheel_8_pbrm_VAL]
  [vdy_Simctrl_tsim] -> Table/1

== system Demo_veDYNA_cs/Vedyna_Vehicle/CPT_MDL/MDL_SW/BrkHyd/System Instance 1/HCI [1,..,n] ==
  Switch : Constant  Value=CPT.MDL_SW.BrkHyd{1}.HCI.Switch.v
  Terminator : Terminator
  tag scope: BrkHyd_1_HCI_SW=global
  wires:
  [BrkHyd_1_HCI_SW] -> Terminator/1
  Switch/1 -> [BrkHyd_1_HCI_SW]

== system Demo_veDYNA_cs/Vedyna_Vehicle/CPT_MDL/MDL_SW/BrkHyd/System Instance 1/pbrmaster [1,..,4] ==
  Switch : Constant  Value=CPT.MDL_SW.BrkHyd{1}.pbrmaster.Switch.v
  Terminator : Terminator
  tag scope: BrkHyd_1_pbrmaster_SW=global
  wires:
  [BrkHyd_1_pbrmaster_SW] -> Terminator/1
  Switch/1 -> [BrkHyd_1_pbrmaster_SW]

== system Demo_veDYNA_cs/Vedyna_Vehicle/CPT_MDL/MDL_SW/Chassis/System Instance 1/HCI [1,..,n] ==
  Switch : Constant  Value=CPT.MDL_SW.Chassis{1}.HCI.Switch.v
  Terminator : Terminator
  tag scope: Chassis_1_HCI_SW=global
  wires:
  [Chassis_1_HCI_SW] -> Terminator/1
  Switch/1 -> [Chassis_1_HCI_SW]

== system Demo_veDYNA_cs/Vedyna_Vehicle/CPT_MDL/MDL_SW/ClutchCtrl/System Instance 1/Clutch [1,..,4] ==
  Switch : Constant  Value=CPT.MDL_SW.ClutchCtrl{1}.Clutch.Switch.v
  Terminator : Terminator
  tag scope: ClutchCtrl_1_Clutch_SW=global
  wires:
  [ClutchCtrl_1_Clutch_SW] -> Terminator/1
  Switch/1 -> [ClutchCtrl_1_Clutch_SW]

== system Demo_veDYNA_cs/Vedyna_Vehicle/CPT_MDL/MDL_SW/ClutchCtrl/System Instance 1/ClutchMode [0,1] ==
  Switch : Constant  Value=CPT.MDL_SW.ClutchCtrl{1}.ClutchMode.Switch.v
  Terminator : Terminator
  tag scope: ClutchCtrl_1_ClutchMode_SW=global
  wires:
  [ClutchCtrl_1_ClutchMode_SW] -> Terminator/1
  Switch/1 -> [ClutchCtrl_1_ClutchMode_SW]

== system Demo_veDYNA_cs/Vedyna_Vehicle/CPT_MDL/MDL_SW/ClutchCtrl/System Instance 1/HCI [1,..,n] ==
  Switch : Constant  Value=CPT.MDL_SW.ClutchCtrl{1}.HCI.Switch.v
  Terminator : Terminator
  tag scope: ClutchCtrl_1_HCI_SW=global
  wires:
  [ClutchCtrl_1_HCI_SW] -> Terminator/1
  Switch/1 -> [ClutchCtrl_1_HCI_SW]

== system Demo_veDYNA_cs/Vedyna_Vehicle/CPT_MDL/MDL_SW/Contact/System Instance 1/RoadZ [1,..,4] ==
  Switch : Constant  Value=CPT.MDL_SW.Contact{1}.RoadZ.Switch.v
  Terminator : Terminator
  tag scope: Contact_1_RoadZ_SW=global
  wires:
  [Contact_1_RoadZ_SW] -> Terminator/1
  Switch/1 -> [Contact_1_RoadZ_SW]

== system Demo_veDYNA_cs/Vedyna_Vehicle/CPT_MDL/MDL_SW/Contact/System Instance 2/RoadZ [1,..,4] ==
  Switch : Constant  Value=CPT.MDL_SW.Contact{2}.RoadZ.Switch.v
  Terminator : Terminator
  tag scope: Contact_2_RoadZ_SW=global
  wires:
  [Contact_2_RoadZ_SW] -> Terminator/1
  Switch/1 -> [Contact_2_RoadZ_SW]

== system Demo_veDYNA_cs/Vedyna_Vehicle/CPT_MDL/MDL_SW/Contact/System Instance 3/RoadZ [1,..,4] ==
  Switch : Constant  Value=CPT.MDL_SW.Contact{3}.RoadZ.Switch.v
  Terminator : Terminator
  tag scope: Contact_3_RoadZ_SW=global
  wires:
  [Contact_3_RoadZ_SW] -> Terminator/1
  Switch/1 -> [Contact_3_RoadZ_SW]

== system Demo_veDYNA_cs/Vedyna_Vehicle/CPT_MDL/MDL_SW/Contact/System Instance 4/RoadZ [1,..,4] ==
  Switch : Constant  Value=CPT.MDL_SW.Contact{4}.RoadZ.Switch.v
  Terminator : Terminator
  tag scope: Contact_4_RoadZ_SW=global
  wires:
  [Contact_4_RoadZ_SW] -> Terminator/1
  Switch/1 -> [Contact_4_RoadZ_SW]

== system Demo_veDYNA_cs/Vedyna_Vehicle/CPT_MDL/MDL_SW/Contact/System Instance 5/RoadZ [1,..,4] ==
  Switch : Constant  Value=CPT.MDL_SW.Contact{5}.RoadZ.Switch.v
  Terminator : Terminator
  tag scope: Contact_5_RoadZ_SW=global
  wires:
  [Contact_5_RoadZ_SW] -> Terminator/1
  Switch/1 -> [Contact_5_RoadZ_SW]

== system Demo_veDYNA_cs/Vedyna_Vehicle/CPT_MDL/MDL_SW/Contact/System Instance 6/RoadZ [1,..,4] ==
  Switch : Constant  Value=CPT.MDL_SW.Contact{6}.RoadZ.Switch.v
  Terminator : Terminator
  tag scope: Contact_6_RoadZ_SW=global
  wires:
  [Contact_6_RoadZ_SW] -> Terminator/1
  Switch/1 -> [Contact_6_RoadZ_SW]

== system Demo_veDYNA_cs/Vedyna_Vehicle/CPT_MDL/MDL_SW/Contact/System Instance 7/RoadZ [1,..,4] ==
  Switch : Constant  Value=CPT.MDL_SW.Contact{7}.RoadZ.Switch.v
  Terminator : Terminator
  tag scope: Contact_7_RoadZ_SW=global
  wires:
  Switch/1 -> [Contact_7_RoadZ_SW]
  [Contact_7_RoadZ_SW] -> Terminator/1

== system Demo_veDYNA_cs/Vedyna_Vehicle/CPT_MDL/MDL_SW/Contact/System Instance 8/RoadZ [1,..,4] ==
  Switch : Constant  Value=CPT.MDL_SW.Contact{8}.RoadZ.Switch.v
  Terminator : Terminator
  tag scope: Contact_8_RoadZ_SW=global
  wires:
  Switch/1 -> [Contact_8_RoadZ_SW]
  [Contact_8_RoadZ_SW] -> Terminator/1

== system Demo_veDYNA_cs/Vedyna_Vehicle/CPT_MDL/MDL_SW/Driveline/System Instance 1/HCI [1,..,n] ==
  Switch : Constant  Value=CPT.MDL_SW.Driveline{1}.HCI.Switch.v
  Terminator : Terminator
  tag scope: Driveline_1_HCI_SW=global
  wires:
  [Driveline_1_HCI_SW] -> Terminator/1
  Switch/1 -> [Driveline_1_HCI_SW]

== system Demo_veDYNA_cs/Vedyna_Vehicle/CPT_MDL/MDL_SW/Driver/System Instance 1/HCI [1,..,n] ==
  Switch : Constant  Value=CPT.MDL_SW.Driver{1}.HCI.Switch.v
  Terminator : Terminator
  tag scope: Driver_1_HCI_SW=global
  wires:
  [Driver_1_HCI_SW] -> Terminator/1
  Switch/1 -> [Driver_1_HCI_SW]

== system Demo_veDYNA_cs/Vedyna_Vehicle/CPT_MDL/MDL_SW/Driver/System Instance 1/acc_comp_scale [1,..,4] ==
  Switch : Constant  Value=CPT.MDL_SW.Driver{1}.acc_comp_scale.Switch.v
  Terminator : Terminator
  tag scope: Driver_1_acc_comp_scale_SW=global
  wires:
  [Driver_1_acc_comp_scale_SW] -> Terminator/1
  Switch/1 -> [Driver_1_acc_comp_scale_SW]

== system Demo_veDYNA_cs/Vedyna_Vehicle/CPT_MDL/MDL_SW/Driver/System Instance 1/adj_acc_gain [1,..,4] ==
  Switch : Constant  Value=CPT.MDL_SW.Driver{1}.adj_acc_gain.Switch.v
  Terminator : Terminator
  tag scope: Driver_1_adj_acc_gain_SW=global
  wires:
  [Driver_1_adj_acc_gain_SW] -> Terminator/1
  Switch/1 -> [Driver_1_adj_acc_gain_SW]

== system Demo_veDYNA_cs/Vedyna_Vehicle/CPT_MDL/MDL_SW/Driver/System Instance 1/adj_brake_gain [1,..,4] ==
  Switch : Constant  Value=CPT.MDL_SW.Driver{1}.adj_brake_gain.Switch.v
  Terminator : Terminator
  tag scope: Driver_1_adj_brake_gain_SW=global
  wires:
  [Driver_1_adj_brake_gain_SW] -> Terminator/1
  Switch/1 -> [Driver_1_adj_brake_gain_SW]

== system Demo_veDYNA_cs/Vedyna_Vehicle/CPT_MDL/MDL_SW/Driver/System Instance 1/ax_min [1,..,4] ==
  Switch : Constant  Value=CPT.MDL_SW.Driver{1}.ax_min.Switch.v
  Terminator : Terminator
  tag scope: Driver_1_ax_min_SW=global
  wires:
  [Driver_1_ax_min_SW] -> Terminator/1
  Switch/1 -> [Driver_1_ax_min_SW]

== system Demo_veDYNA_cs/Vedyna_Vehicle/CPT_MDL/MDL_SW/Driver/System Instance 1/ctrl_acc_smooth_t [1,..,4] ==
  Switch : Constant  Value=CPT.MDL_SW.Driver{1}.ctrl_acc_smooth_t.Switch.v
  Terminator : Terminator
  tag scope: Driver_1_ctrl_acc_smooth_t_SW=global
  wires:
  [Driver_1_ctrl_acc_smooth_t_SW] -> Terminator/1
  Switch/1 -> [Driver_1_ctrl_acc_smooth_t_SW]

== system Demo_veDYNA_cs/Vedyna_Vehicle/CPT_MDL/MDL_SW/Driver/System Instance 1/cu_comp_scale [1,..,4] ==
  Switch : Constant  Value=CPT.MDL_SW.Driver{1}.cu_comp_scale.Switch.v
  Terminator : Terminator
  tag scope: Driver_1_cu_comp_scale_SW=global
  wires:
  [Driver_1_cu_comp_scale_SW] -> Terminator/1
  Switch/1 -> [Driver_1_cu_comp_scale_SW]

== system Demo_veDYNA_cs/Vedyna_Vehicle/CPT_MDL/MDL_SW/Driver/System Instance 1/cu_path [1,..,4] ==
  Switch : Constant  Value=CPT.MDL_SW.Driver{1}.cu_path.Switch.v
  Terminator : Terminator
  tag scope: Driver_1_cu_path_SW=global
  wires:
  [Driver_1_cu_path_SW] -> Terminator/1
  Switch/1 -> [Driver_1_cu_path_SW]

== system Demo_veDYNA_cs/Vedyna_Vehicle/CPT_MDL/MDL_SW/Driver/System Instance 1/front_stiff [1,..,4] ==
  Switch : Constant  Value=CPT.MDL_SW.Driver{1}.front_stiff.Switch.v
  Terminator : Terminator
  tag scope: Driver_1_front_stiff_SW=global
  wires:
  [Driver_1_front_stiff_SW] -> Terminator/1
  Switch/1 -> [Driver_1_front_stiff_SW]

== system Demo_veDYNA_cs/Vedyna_Vehicle/CPT_MDL/MDL_SW/Driver/System Instance 1/front_stiff_sw [1,..,4] ==
  Switch : Constant  Value=CPT.MDL_SW.Driver{1}.front_stiff_sw.Switch.v
  Terminator : Terminator
  tag scope: Driver_1_front_stiff_sw_SW=global
  wires:
  [Driver_1_front_stiff_sw_SW] -> Terminator/1
  Switch/1 -> [Driver_1_front_stiff_sw_SW]

== system Demo_veDYNA_cs/Vedyna_Vehicle/CPT_MDL/MDL_SW/Driver/System Instance 1/gain_lat [1,..,4] ==
  Switch : Constant  Value=CPT.MDL_SW.Driver{1}.gain_lat.Switch.v
  Terminator : Terminator
  tag scope: Driver_1_gain_lat_SW=global
  wires:
  [Driver_1_gain_lat_SW] -> Terminator/1
  Switch/1 -> [Driver_1_gain_lat_SW]

== system Demo_veDYNA_cs/Vedyna_Vehicle/CPT_MDL/MDL_SW/Driver/System Instance 1/gain_long [1,..,4] ==
  Switch : Constant  Value=CPT.MDL_SW.Driver{1}.gain_long.Switch.v
  Terminator : Terminator
  tag scope: Driver_1_gain_long_SW=global
  wires:
  [Driver_1_gain_long_SW] -> Terminator/1
  Switch/1 -> [Driver_1_gain_long_SW]

== system Demo_veDYNA_cs/Vedyna_Vehicle/CPT_MDL/MDL_SW/Driver/System Instance 1/lat_for_r_scale [1,..,4] ==
  Switch : Constant  Value=CPT.MDL_SW.Driver{1}.lat_for_r_scale.Switch.v
  Terminator : Terminator
  tag scope: Driver_1_lat_for_r_scale_SW=global
  wires:
  [Driver_1_lat_for_r_scale_SW] -> Terminator/1
  Switch/1 -> [Driver_1_lat_for_r_scale_SW]

== system Demo_veDYNA_cs/Vedyna_Vehicle/CPT_MDL/MDL_SW/Driver/System Instance 1/lat_for_r_smooth_t [1,..,4] ==
  Switch : Constant  Value=CPT.MDL_SW.Driver{1}.lat_for_r_smooth_t.Switch.v
  Terminator : Terminator
  tag scope: Driver_1_lat_for_r_smooth_t_SW=global
  wires:
  [Driver_1_lat_for_r_smooth_t_SW] -> Terminator/1
  Switch/1 -> [Driver_1_lat_for_r_smooth_t_SW]
